simulink model "iopid"  (R2021b)
settings: Solver=FixedStepDiscrete  StartTime=0.0  StopTime=100e-3  RelTol=1e-3
Description:
  | Symmetric FIR Filter
  | This example shows how to use HDL Coder(TM) to check, generate,
  | and verify HDL for a fixed-point symmetric FIR filter.
settings Model: DataTypeOverride=Off  Creator=The MathWorks, Inc.  LastModifiedBy=Marco Milanesi
settings SolverCC: AlgebraicLoopSolver=TrustRegion  AutoInsertRateTranBlk=on
settings DataIOCC: LimitDataPoints=on  SaveFormat=Array  SaveOutput=off  SignalLogging=off  SaveTime=off  ReturnWorkspaceOutputs=off  SignalLoggingName=logsOut
settings OptimizationCC: BlockReduction=off  BooleanDataType=off  ConditionallyExecuteInputs=off  DefaultParameterBehavior=Inlined  InheritOutputTypeSmallerThanSingle=on  InlineInvariantSignals=on  ExpressionDepthLimit=2147483647  InitFltsAndDblsToZero=on  LifeSpan=inf  BufferReusableBoundary=off
settings DebuggingCC: AlgebraicLoopMsg=error  SaveWithParameterizedLinksMsg=none  UnderspecifiedInitializationDetection=Classic  MergeDetectMultiDrivingBlocksExec=none  CheckExecutionContextPreStartOutputMsg=on  SignalResolutionControl=TryResolveAllWithWarning  MultiTaskDSMMsg=warning  MultiTaskCondExecSysMsg=none  SingleTaskRateTransMsg=error  IntegerOverflowMsg=none  ParameterPrecisionLossMsg=none  FcnCallInpInsideContextMsg=warning  BusObjectLabelMismatch=none  StateNameClashWarn=warning  SFUnexpectedBacktrackingDiag=warning  SFNoUnconditionalDefaultTransitionDiag=warning  SFExecutionAtInitializationDiag=none  SFMachineParentedDataDiag=warning  IntegerSaturationMsg=none  ArithmeticOperatorsInVariantConditions=warning
settings HardwareCC: ProdBitPerPointer=32  ProdBitPerSizeT=32  ProdBitPerPtrDiffT=32  ProdLargestAtomicFloat=None  ProdIntDivRoundTo=Undefined  ProdEndianess=Unspecified  ProdWordSize=32  ProdHWDeviceType=ASIC/FPGA  TargetUnknown=on  ProdEqTarget=off
settings ModelReferenceCC: PropagateSignalLabelsOutOfModel=off
settings SFSimCC: SimUseLocalCustomCode=off  CustomCodeUndefinedFunction=UseInterfaceOnly
settings RTWCC: RTWUseLocalCustomCode=off
settings CodeAppCC: StateflowObjectComments=on
settings GRTTargetCC: TargetFcnLib=ansi_tfl_tmw.mat  TargetLangStandard=C89/C90 (ANSI)  CombineOutputUpdateFcns=off  GRTInterface=on
settings ConfigComp: CovMetricSettings=dw  CovSaveCumulativeToWorkspaceVar=on  CovSaveSingleToWorkspaceVar=on  CovExternalEMLEnable=off

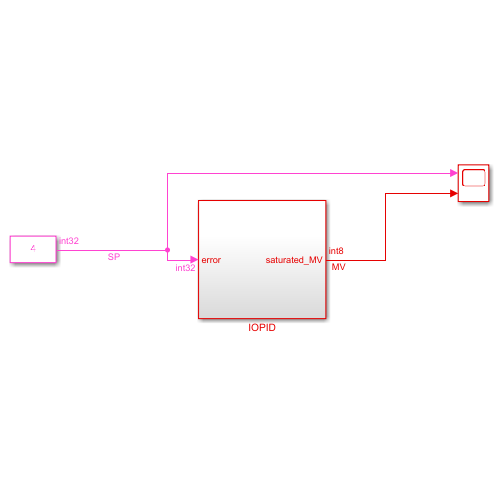
[thumbnail: Simulink's stored preview of the top-level diagram]
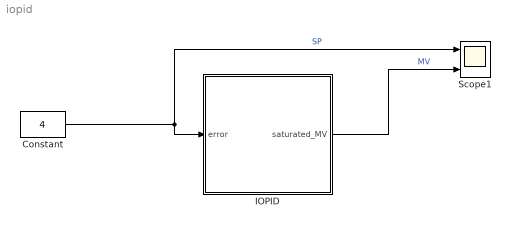
== system iopid ==
  Constant : Constant  Value=4  OutDataTypeStr=fixdt(1,32,0)
  IOPID : Subsystem
  Scope1 : Scope  NumInputPorts=2
  wires:
  Constant/1 -> Scope1/1, IOPID/1(error)  "SP"
  IOPID/1(saturated_MV) -> Scope1/2  "MV"

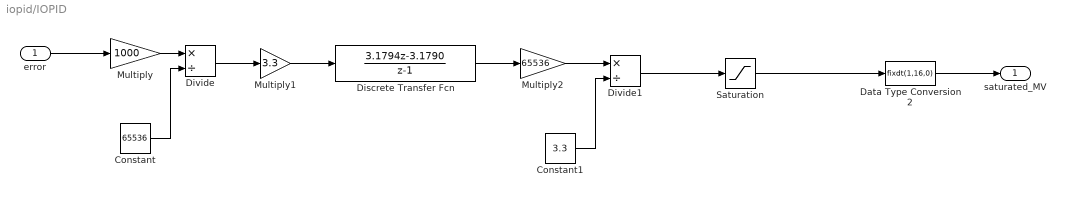
== system iopid/IOPID ==
  error : Inport  OutDataTypeStr=fixdt(1,32,0)  SampleTime=80e-9
  Constant : Constant  Value=65536  OutDataTypeStr=fixdt(1,32,0)
  Constant1 : Constant  Value=3.3  OutDataTypeStr=fixdt(1,32,0)
  Data Type Conversion2 : DataTypeConversion  OutDataTypeStr=fixdt(1,16,0)
  Discrete Transfer Fcn : DiscreteTransferFcn  Numerator=[3.1794 -3.1790]  Denominator=[1 -1]  SampleTime=80e-9  NumCoefDataTypeStr=fixdt(1,32,0)  DenCoefDataTypeStr=fixdt(1,32,0)  NumProductDataTypeStr=fixdt(1,32,0)  DenProductDataTypeStr=fixdt(1,32,0)  NumAccumDataTypeStr=fixdt(1,32,0)  DenAccumDataTypeStr=fixdt(1,32,0)  OutDataTypeStr=fixdt(1,32,0)
  Divide : Product  Inputs=*/  OutDataTypeStr=fixdt(1,32,0)  RndMeth=Zero  SaturateOnIntegerOverflow=on
  Divide1 : Product  Inputs=*/  OutDataTypeStr=fixdt(1,32,0)  RndMeth=Zero  SaturateOnIntegerOverflow=on
  Multiply : Gain  Gain=1000  OutDataTypeStr=fixdt(1,32,0)
  Multiply1 : Gain  Gain=3.3  OutDataTypeStr=fixdt(1,32,0)
  Multiply2 : Gain  Gain=65536  OutDataTypeStr=fixdt(1,32,0)
  Saturation : Saturate  UpperLimit=255  LowerLimit=0  OutDataTypeStr=fixdt(1,32,0)
  saturated_MV : Outport  OutDataTypeStr=fixdt(1,16,0)  SampleTime=80e-9  VectorParamsAs1DForOutWhenUnconnected=off
  wires:
  Data Type Conversion2/1 -> saturated_MV/1
  Saturation/1 -> Data Type Conversion2/1
  error/1 -> Multiply/1
  Multiply/1 -> Divide/1
  Constant/1 -> Divide/2
  Divide/1 -> Multiply1/1
  Multiply1/1 -> Discrete Transfer Fcn/1
  Discrete Transfer Fcn/1 -> Multiply2/1
  Constant1/1 -> Divide1/2
  Multiply2/1 -> Divide1/1
  Divide1/1 -> Saturation/1
